simulink model "motorcycle_plant"  (R2018b)
settings: Solver=VariableStepAuto  StartTime=0.0  StopTime=10.0  RelTol=1e-3
values from neighbouring files (symbols this model uses):
  delta_i = 0    [parameters.m]
  epsilon = 27.72*pi/180    (= 0.483805268653)    [parameters.m]
  J_s = 0.41    [parameters.m]
  J_z = 40    [parameters.m]
  k_af = 12.36    [parameters.m]
  k_ar = 11    [parameters.m]
  l_f = 0.5    [parameters.m]
  l_r = 0.5    [parameters.m]
  N_f = M*g/2    (= 1343.97)    [parameters.m]
  N_r = M*g/2    (= 1343.97)    [parameters.m]
  t_n = r*sin(epsilon)    [parameters.m]
settings Model: Creator=Master Broda  LastModifiedBy=Master Broda

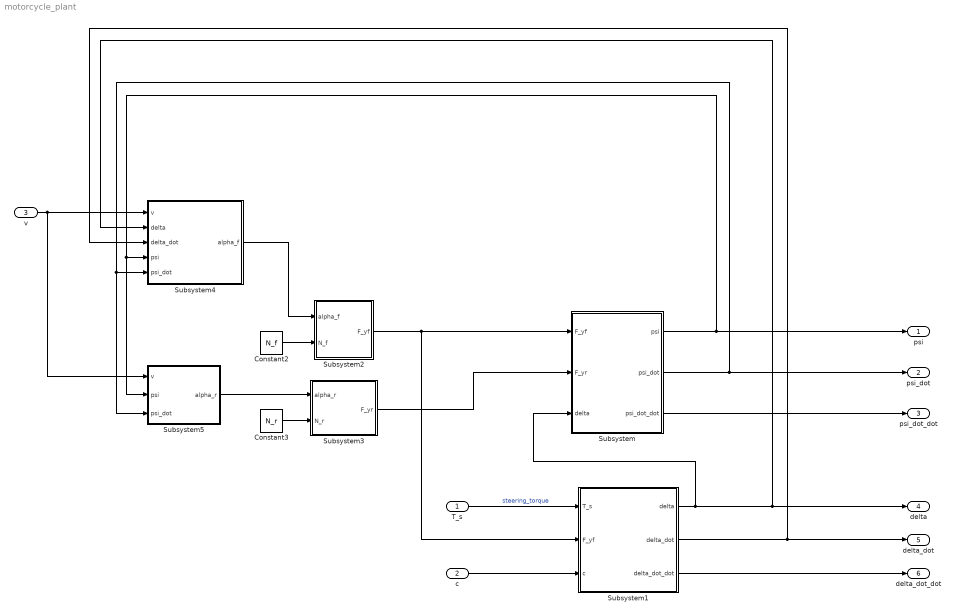
== system motorcycle_plant ==
  "T_s " : Inport
  "c " : Inport  Port=2
  v : Inport  Port=3
  Constant2 : Constant  Value=N_f
  Constant3 : Constant  Value=N_r
  Subsystem : Subsystem
  Subsystem1 : Subsystem
  Subsystem2 : Subsystem
  Subsystem3 : Subsystem
  Subsystem4 : Subsystem
  Subsystem5 : Subsystem
  psi : Outport
  psi_dot : Outport  Port=2
  psi_dot_dot : Outport  Port=3
  delta : Outport  Port=4
  delta_dot : Outport  Port=5
  delta_dot_dot : Outport  Port=6
  wires:
  "T_s "/1 -> Subsystem1/1("T_s ")  "steering_torque"
  Subsystem2/1("F_yf ") -> Subsystem1/2("F_yf "), Subsystem/1("F_yf ")
  "c "/1 -> Subsystem1/3("c ")
  Subsystem1/3(delta_dot_dot) -> delta_dot_dot/1
  Subsystem3/1(F_yr) -> Subsystem/2("F_yr ")
  Constant2/1 -> Subsystem2/2("N_f ")
  Constant3/1 -> Subsystem3/2(N_r)
  Subsystem/1("psi ") -> psi/1, Subsystem4/4(psi), Subsystem5/2(psi)
  Subsystem/3("psi_dot_dot ") -> psi_dot_dot/1
  Subsystem4/1("alpha_f ") -> Subsystem2/1(alpha_f)
  Subsystem5/1(alpha_r) -> Subsystem3/1("alpha_r ")
  v/1 -> Subsystem4/1("v "), Subsystem5/1(v)
  Subsystem/2("psi_dot ") -> psi_dot/1, Subsystem4/5(psi_dot), Subsystem5/3(psi_dot)
  Subsystem1/1("delta ") -> delta/1, Subsystem4/2(delta), Subsystem/3(delta)
  Subsystem1/2(delta_dot) -> delta_dot/1, Subsystem4/3(delta_dot)

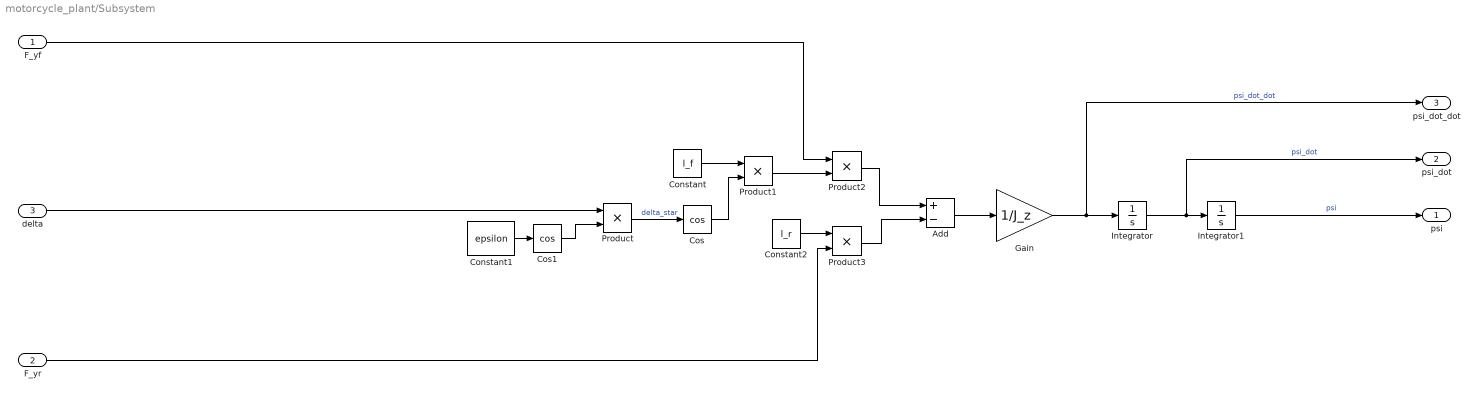
== system motorcycle_plant/Subsystem ==
  "F_yf " : Inport
  "F_yr " : Inport  Port=2
  delta : Inport  Port=3
  Add : Sum  Inputs=+-
  Constant : Constant  Value=l_f
  Constant1 : Constant  Value=epsilon
  Constant2 : Constant  Value=l_r
  Cos : Trigonometry  Operator=cos
  Cos1 : Trigonometry  Operator=cos
  Gain : Gain  Gain=1/J_z
  Integrator : Integrator
  Integrator1 : Integrator
  Product{,1..3} (4 alike) : Product
  "psi " : Outport
  "psi_dot " : Outport  Port=2
  "psi_dot_dot " : Outport  Port=3
  wires:
  delta/1 -> Product/1
  Integrator/1 -> "psi_dot "/1, Integrator1/1  "psi_dot"
  Cos1/1 -> Product/2
  Constant/1 -> Product1/1
  Constant2/1 -> Product3/1
  Constant1/1 -> Cos1/1
  Gain/1 -> "psi_dot_dot "/1, Integrator/1  "psi_dot_dot"
  Product/1 -> Cos/1  "delta_star"
  Cos/1 -> Product1/2
  Product1/1 -> Product2/2
  Integrator1/1 -> "psi "/1  "psi"
  Product3/1 -> Add/2
  "F_yr "/1 -> Product3/2
  "F_yf "/1 -> Product2/1
  Product2/1 -> Add/1
  Add/1 -> Gain/1

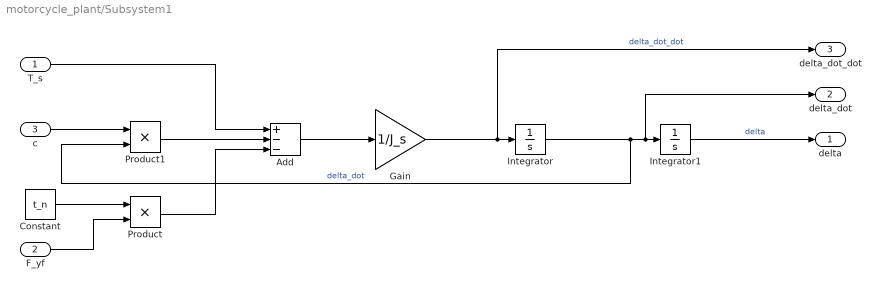
== system motorcycle_plant/Subsystem1 ==
  "T_s " : Inport
  "F_yf " : Inport  Port=2
  "c " : Inport  Port=3
  Add : Sum  Inputs=+--
  Constant : Constant  Value=t_n
  Gain : Gain  Gain=1/J_s
  Integrator : Integrator
  Integrator1 : Integrator  InitialCondition=delta_i
  Product : Product
  Product1 : Product
  "delta " : Outport
  delta_dot : Outport  Port=2
  delta_dot_dot : Outport  Port=3
  wires:
  Integrator1/1 -> "delta "/1  "delta"
  Constant/1 -> Product/1
  Integrator/1 -> Product1/2, delta_dot/1, Integrator1/1  "delta_dot"
  "T_s "/1 -> Add/1
  Gain/1 -> delta_dot_dot/1, Integrator/1  "delta_dot_dot"
  Product1/1 -> Add/2
  Add/1 -> Gain/1
  Product/1 -> Add/3
  "c "/1 -> Product1/1
  "F_yf "/1 -> Product/2

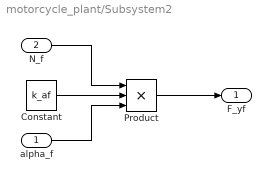
== system motorcycle_plant/Subsystem2 ==
  alpha_f : Inport
  "N_f " : Inport  Port=2
  Constant : Constant  Value=k_af
  Product : Product  Inputs=3
  "F_yf " : Outport
  wires:
  Constant/1 -> Product/2
  alpha_f/1 -> Product/3
  "N_f "/1 -> Product/1
  Product/1 -> "F_yf "/1

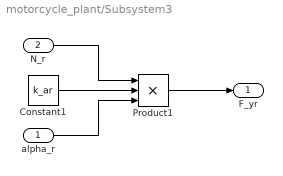
== system motorcycle_plant/Subsystem3 ==
  "alpha_r " : Inport
  N_r : Inport  Port=2
  Constant1 : Constant  Value=k_ar
  Product1 : Product  Inputs=3
  F_yr : Outport
  wires:
  "alpha_r "/1 -> Product1/3
  Product1/1 -> F_yr/1
  Constant1/1 -> Product1/2
  N_r/1 -> Product1/1

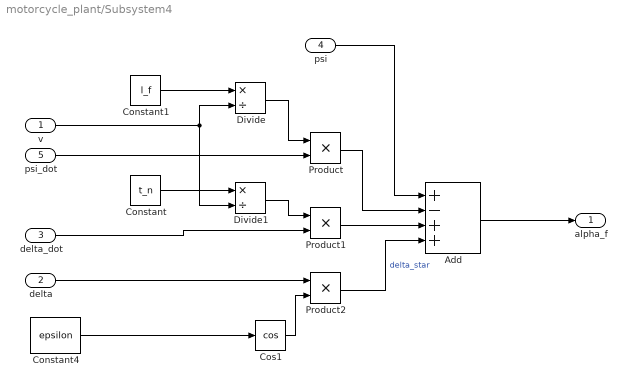
== system motorcycle_plant/Subsystem4 ==
  "v " : Inport
  delta : Inport  Port=2
  delta_dot : Inport  Port=3
  psi : Inport  Port=4
  psi_dot : Inport  Port=5
  Add : Sum  Inputs=+-++
  Constant : Constant  Value=t_n  VectorParams1D=off
  Constant1 : Constant  Value=l_f  VectorParams1D=off
  Constant4 : Constant  Value=epsilon
  Cos1 : Trigonometry  Operator=cos
  Divide : Product  Inputs=*/
  Divide1 : Product  Inputs=*/
  Product : Product
  Product1 : Product
  Product2 : Product
  "alpha_f " : Outport
  wires:
  Product1/1 -> Add/3
  Cos1/1 -> Product2/2
  Divide1/1 -> Product1/1
  Constant1/1 -> Divide/1
  Divide/1 -> Product/1
  psi_dot/1 -> Product/2
  Add/1 -> "alpha_f "/1
  Constant/1 -> Divide1/1
  delta_dot/1 -> Product1/2
  Product2/1 -> Add/4  "delta_star"
  Product/1 -> Add/2
  delta/1 -> Product2/1
  Constant4/1 -> Cos1/1
  "v "/1 -> Divide1/2, Divide/2
  psi/1 -> Add/1

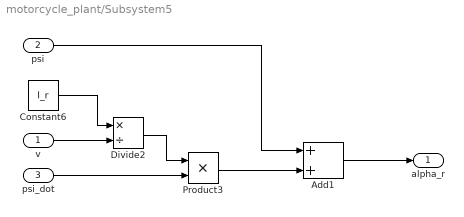
== system motorcycle_plant/Subsystem5 ==
  v : Inport
  psi : Inport  Port=2
  psi_dot : Inport  Port=3
  Add1 : Sum
  Constant6 : Constant  Value=l_r  VectorParams1D=off
  Divide2 : Product  Inputs=*/
  Product3 : Product
  alpha_r : Outport
  wires:
  psi_dot/1 -> Product3/2
  Divide2/1 -> Product3/1
  v/1 -> Divide2/2
  Product3/1 -> Add1/2
  Add1/1 -> alpha_r/1
  psi/1 -> Add1/1
  Constant6/1 -> Divide2/1
